simulink model "Modelo_MV_CIGRE_IPSD"  (R2019b)
settings: Solver=FixedStepAuto  StartTime=0.0  StopTime=0.3  FixedStep=Ts  RelTol=1e-3
PreLoadFcn:
  | r_1=0.501
  | l_1=0.716/(60*2*pi)
  | c_1=10e-6/(60*2*pi)
  | r_0=0.817
  | l_0=1.598 /(60*2*pi)
  | c_0=10e-6/(60*2*pi)
  | Sb=50e6
  | Ts=1e-4
InitFcn:
  | r_1=0.501;
  | l_1=0.716/(60*2*pi);
  | c_1=10e-6/(60*2*pi);
  | r_0=0.817;
  | l_0=1.598 /(60*2*pi);
  | c_0=10e-6/(60*2*pi);
  | Sb=50e6;
  | Ts=1e-4;
StartFcn:
  | r_1=0.501
  | l_1=0.716/(60*2*pi)
  | c_1=10e-6/(60*2*pi)
  | r_0=0.817
  | l_0=1.598 /(60*2*pi)
  | c_0=10e-6/(60*2*pi)
  | Sb=50e6
  | Ts=1e-5
undefined symbols (not defined in the file): D1, Delta
libraries: powerlib_meascontrol x112, powerlib x55, simulink x6
(part 2 of 3)

== system Modelo_MV_CIGRE_IPSD/DER1 ==
  Control IBRs : Subsystem
  Controlled Voltage Source : powerlib/Electrical Sources/Controlled Voltage Source  Initialize=on  Source_Type=AC  Amplitude=400*sqrt(2/3)  Phase=0  Frequency=60  Measurements=None
      settings: SourceProductName=Simscape Electrical
  Controlled Voltage Source2 : powerlib/Electrical Sources/Controlled Voltage Source  Initialize=on  Source_Type=AC  Amplitude=400*sqrt(2/3)  Phase=120  Frequency=60  Measurements=None
      settings: SourceProductName=Simscape Electrical
  Controlled Voltage Source3 : powerlib/Electrical Sources/Controlled Voltage Source  Initialize=on  Source_Type=AC  Amplitude=400*sqrt(2/3)  Phase=-120  Frequency=60  Measurements=None
      settings: SourceProductName=Simscape Electrical
  Ground : powerlib/Elements/Ground  LConnTagsString=a
      settings: SourceProductName=Simscape Electrical
  "Power (3ph, Instantaneous)" : powerlib_meascontrol/Measurements/Power (3ph, Instantaneous)
      settings: SourceProductName=Simscape Electrical
  Scope : Scope
  Scope1 : Scope  NumInputPorts=2
  Scope4 : Scope  NumInputPorts=3
  Scope5 : Scope
  Scope6 : Scope
  Three-Phase Series RLC Branch1 : powerlib/Elements/Three-Phase Series RLC Branch  LConnTagsString=A|B|C  RConnTagsString=A|B|C  BranchType=RL  Resistance=0.57  Inductance=1.5e-3  Capacitance=1e-6  Measurements=None
      settings: SourceProductName=Simscape Electrical
  Three-Phase Series RLC Branch2 : powerlib/Elements/Three-Phase Series RLC Branch  LConnTagsString=A|B|C  RConnTagsString=A|B|C  BranchType=C  Resistance=0.01  Inductance=1e-3  Capacitance=3e-6  Measurements=None
      settings: SourceProductName=Simscape Electrical
  Three-Phase V-I Measurement : powerlib/Measurements/Three-Phase V-I Measurement  VoltageMeasurement=phase-to-ground  SetLabelV=on  LabelV=Vabc_DER2  Vpu=on  VpuLL=off  CurrentMeasurement=yes  SetLabelI=on  LabelI=Iabc_DER2  Ipu=on  Pbase=100e3  Vbase=400  OutputType=Complex  PhasorSimulation=off  PSBequivalent=0
      settings: SourceProductName=Simscape Electrical
  Three-Phase Transformer Inductance Matrix Type (Two Windings) : powerlib/Elements/Three-Phase Transformer Inductance Matrix Type (Two Windings)  CoreType=Three single-phase cores  Winding1Connection=Yg  Winding2Connection=Delta (D1)  AutoTransformer=off  Measurements=None  NominalPower=[150e3, 60]  VLLnom=[20e3, 400]  WindingResistances=[0.01, 0.01]  NoLoadIexcPos=2  NoLoadPlossPos=1000  ShortCircuitReactancePos=0.06  ShortCircuitReactancePosAuto=0.06  NoLoadIexcZero=100  NoLoadPlossZero=1500  ShortCircuitReactanceZero=0.03  ShortCircuitReactanceZeroAuto=0.03
      settings: SourceProductName=Simscape Electrical  SourceProductBaseCode=PS
  A : PMIOPort  Side=Left
  B : PMIOPort  Port=2  Side=Left
  C : PMIOPort  Port=3  Side=Left
  wires:
  Control IBRs/2(Vb) -> Scope4/2, Controlled Voltage Source2/1
  [Vabc_DER2] -> "Power (3ph, Instantaneous)"/1, Scope/1, Scope1/2, Control IBRs/1(Vmeas)
  Control IBRs/3(Vc) -> Scope4/3, Controlled Voltage Source3/1
  "Power (3ph, Instantaneous)"/1 -> Scope5/1
  Control IBRs/1(Va) -> Scope4/1, Controlled Voltage Source/1
  "Power (3ph, Instantaneous)"/2 -> Scope6/1
  [Iabc_DER2] -> Scope1/1, "Power (3ph, Instantaneous)"/2, Control IBRs/2(Imeas)
  connections:
  Ground/LConn1 -- Three-Phase Series RLC Branch2/RConn1 -- Three-Phase Series RLC Branch2/RConn3 -- Controlled Voltage Source/LConn1 -- Controlled Voltage Source2/LConn1 -- Controlled Voltage Source3/LConn1 -- Three-Phase Series RLC Branch2/RConn2
  C/RConn1 -- Three-Phase Transformer Inductance Matrix Type (Two Windings)/LConn3
  Three-Phase Series RLC Branch1/RConn1 -- Controlled Voltage Source/RConn1
  Three-Phase Transformer Inductance Matrix Type (Two Windings)/RConn3 -- Three-Phase V-I Measurement/RConn3
  Three-Phase Transformer Inductance Matrix Type (Two Windings)/LConn2 -- B/RConn1
  Three-Phase Series RLC Branch1/LConn3 -- Three-Phase V-I Measurement/LConn3 -- Three-Phase Series RLC Branch2/LConn3
  Three-Phase Series RLC Branch1/RConn2 -- Controlled Voltage Source2/RConn1
  Three-Phase Series RLC Branch1/LConn1 -- Three-Phase V-I Measurement/LConn1 -- Three-Phase Series RLC Branch2/LConn1
  Three-Phase V-I Measurement/RConn1 -- Three-Phase Transformer Inductance Matrix Type (Two Windings)/RConn1
  Three-Phase V-I Measurement/RConn2 -- Three-Phase Transformer Inductance Matrix Type (Two Windings)/RConn2
  Three-Phase Series RLC Branch1/RConn3 -- Controlled Voltage Source3/RConn1
  Three-Phase Series RLC Branch1/LConn2 -- Three-Phase Series RLC Branch2/LConn2 -- Three-Phase V-I Measurement/LConn2
  A/RConn1 -- Three-Phase Transformer Inductance Matrix Type (Two Windings)/LConn1

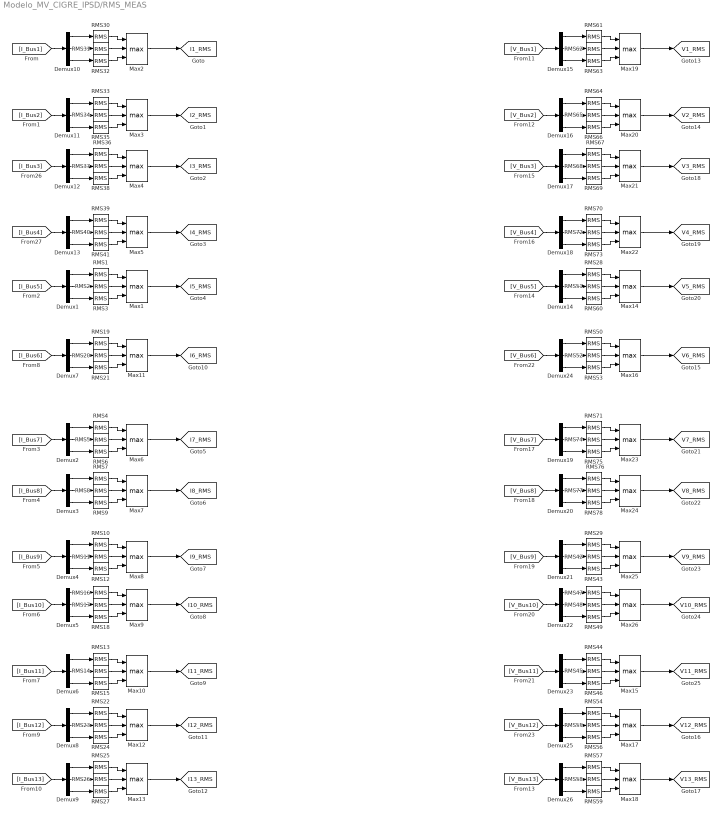
== system Modelo_MV_CIGRE_IPSD/RMS_MEAS ==
  Demux{1..26} (26 alike) : Demux  Outputs=3
  Max{1..26} (26 alike) : MinMax  Function=max  Inputs=3
  RMS{1..78} (78 alike) : powerlib_meascontrol/Measurements/RMS  TrueRMS=on  Freq=60  RMSInit=120  Ts=0
      settings: SourceProductName=Simscape Electrical
  tag scope: I10_RMS=global, I11_RMS=global, I12_RMS=global, I13_RMS=global, I1_RMS=global, I2_RMS=global, I3_RMS=global, I4_RMS=global, I5_RMS=global, I6_RMS=global, I7_RMS=global, I8_RMS=global, I9_RMS=global, V10_RMS=global, V11_RMS=global, V12_RMS=global, V13_RMS=global, V1_RMS=global, V2_RMS=global, V3_RMS=global, V4_RMS=global, V5_RMS=global, V6_RMS=global, V7_RMS=global, V8_RMS=global, V9_RMS=global
  wires:
  Demux10/3 -> RMS32/1
  RMS32/1 -> Max2/3
  RMS34/1 -> Max3/2
  RMS41/1 -> Max5/3
  RMS31/1 -> Max2/2
  Demux11/3 -> RMS35/1
  Demux10/1 -> RMS30/1
  [I_Bus1] -> Demux10/1
  Demux13/2 -> RMS40/1
  Demux12/2 -> RMS37/1
  Demux10/2 -> RMS31/1
  RMS35/1 -> Max3/3
  Demux11/2 -> RMS34/1
  RMS30/1 -> Max2/1
  [I_Bus2] -> Demux11/1
  Demux13/1 -> RMS39/1
  [I_Bus4] -> Demux13/1
  Demux11/1 -> RMS33/1
  RMS33/1 -> Max3/1
  RMS40/1 -> Max5/2
  Demux12/1 -> RMS36/1
  RMS36/1 -> Max4/1
  RMS37/1 -> Max4/2
  RMS39/1 -> Max5/1
  Demux13/3 -> RMS41/1
  RMS38/1 -> Max4/3
  [I_Bus3] -> Demux12/1
  Demux12/3 -> RMS38/1
  Demux3/3 -> RMS9/1
  [I_Bus8] -> Demux3/1
  RMS9/1 -> Max7/3
  Demux4/3 -> RMS12/1
  RMS10/1 -> Max8/1
  RMS8/1 -> Max7/2
  RMS7/1 -> Max7/1
  Demux3/1 -> RMS7/1
  RMS11/1 -> Max8/2
  RMS4/1 -> Max6/1
  Demux2/1 -> RMS4/1
  [I_Bus9] -> Demux4/1
  Demux4/1 -> RMS10/1
  [I_Bus7] -> Demux2/1
  RMS1/1 -> Max1/1
  Demux2/2 -> RMS5/1
  RMS6/1 -> Max6/3
  Demux1/2 -> RMS2/1
  Demux3/2 -> RMS8/1
  Demux4/2 -> RMS11/1
  [I_Bus5] -> Demux1/1
  Demux1/1 -> RMS1/1
  Demux2/3 -> RMS6/1
  RMS2/1 -> Max1/2
  RMS12/1 -> Max8/3
  RMS5/1 -> Max6/2
  RMS3/1 -> Max1/3
  Demux1/3 -> RMS3/1
  RMS15/1 -> Max10/3
  Demux6/2 -> RMS14/1
  Demux5/2 -> RMS17/1
  Demux6/1 -> RMS13/1
  [I_Bus11] -> Demux6/1
  RMS14/1 -> Max10/2
  Demux5/1 -> RMS16/1
  RMS16/1 -> Max9/1
  RMS17/1 -> Max9/2
  RMS13/1 -> Max10/1
  Demux6/3 -> RMS15/1
  RMS18/1 -> Max9/3
  [I_Bus10] -> Demux5/1
  Demux5/3 -> RMS18/1
  Max2/1 -> [I1_RMS]
  Max3/1 -> [I2_RMS]
  Max4/1 -> [I3_RMS]
  Max5/1 -> [I4_RMS]
  Max1/1 -> [I5_RMS]
  Max6/1 -> [I7_RMS]
  Max7/1 -> [I8_RMS]
  Max8/1 -> [I9_RMS]
  Max9/1 -> [I10_RMS]
  Max10/1 -> [I11_RMS]
  Max11/1 -> [I6_RMS]
  Demux7/3 -> RMS21/1
  RMS21/1 -> Max11/3
  RMS20/1 -> Max11/2
  Demux7/1 -> RMS19/1
  [I_Bus6] -> Demux7/1
  Demux7/2 -> RMS20/1
  RMS19/1 -> Max11/1
  Max12/1 -> [I12_RMS]
  Demux8/3 -> RMS24/1
  RMS22/1 -> Max12/1
  RMS23/1 -> Max12/2
  [I_Bus12] -> Demux8/1
  Demux8/1 -> RMS22/1
  Demux8/2 -> RMS23/1
  RMS24/1 -> Max12/3
  RMS27/1 -> Max13/3
  Demux9/2 -> RMS26/1
  Demux9/1 -> RMS25/1
  [I_Bus13] -> Demux9/1
  RMS26/1 -> Max13/2
  RMS25/1 -> Max13/1
  Demux9/3 -> RMS27/1
  Max13/1 -> [I13_RMS]
  Max18/1 -> [V13_RMS]
  Demux26/3 -> RMS59/1
  RMS57/1 -> Max18/1
  RMS58/1 -> Max18/2
  [V_Bus13] -> Demux26/1
  Demux26/1 -> RMS57/1
  Demux26/2 -> RMS58/1
  RMS59/1 -> Max18/3
  RMS56/1 -> Max17/3
  Demux25/2 -> RMS55/1
  Demux25/1 -> RMS54/1
  [V_Bus12] -> Demux25/1
  RMS55/1 -> Max17/2
  RMS54/1 -> Max17/1
  Demux25/3 -> RMS56/1
  Max17/1 -> [V12_RMS]
  RMS50/1 -> Max16/1
  Demux24/2 -> RMS52/1
  [V_Bus6] -> Demux24/1
  Demux24/1 -> RMS50/1
  RMS52/1 -> Max16/2
  RMS53/1 -> Max16/3
  Demux24/3 -> RMS53/1
  Max16/1 -> [V6_RMS]
  Max15/1 -> [V11_RMS]
  Max26/1 -> [V10_RMS]
  Max25/1 -> [V9_RMS]
  Max24/1 -> [V8_RMS]
  Max23/1 -> [V7_RMS]
  Max14/1 -> [V5_RMS]
  Max22/1 -> [V4_RMS]
  Max21/1 -> [V3_RMS]
  Max20/1 -> [V2_RMS]
  Max19/1 -> [V1_RMS]
  Demux22/3 -> RMS49/1
  [V_Bus10] -> Demux22/1
  RMS49/1 -> Max26/3
  Demux23/3 -> RMS46/1
  RMS44/1 -> Max15/1
  RMS48/1 -> Max26/2
  RMS47/1 -> Max26/1
  Demux22/1 -> RMS47/1
  RMS45/1 -> Max15/2
  [V_Bus11] -> Demux23/1
  Demux23/1 -> RMS44/1
  Demux22/2 -> RMS48/1
  Demux23/2 -> RMS45/1
  RMS46/1 -> Max15/3
  Demux14/3 -> RMS60/1
  RMS60/1 -> Max14/3
  RMS74/1 -> Max23/2
  RMS43/1 -> Max25/3
  RMS51/1 -> Max14/2
  Demux19/3 -> RMS75/1
  Demux14/1 -> RMS28/1
  [V_Bus5] -> Demux14/1
  Demux21/2 -> RMS42/1
  Demux20/2 -> RMS77/1
  Demux14/2 -> RMS51/1
  RMS75/1 -> Max23/3
  Demux19/2 -> RMS74/1
  RMS28/1 -> Max14/1
  [V_Bus7] -> Demux19/1
  Demux21/1 -> RMS29/1
  [V_Bus9] -> Demux21/1
  Demux19/1 -> RMS71/1
  RMS71/1 -> Max23/1
  RMS42/1 -> Max25/2
  Demux20/1 -> RMS76/1
  RMS76/1 -> Max24/1
  RMS77/1 -> Max24/2
  RMS29/1 -> Max25/1
  Demux21/3 -> RMS43/1
  RMS78/1 -> Max24/3
  [V_Bus8] -> Demux20/1
  Demux20/3 -> RMS78/1
  Demux17/3 -> RMS69/1
  [V_Bus3] -> Demux17/1
  RMS69/1 -> Max21/3
  Demux18/3 -> RMS73/1
  RMS70/1 -> Max22/1
  RMS68/1 -> Max21/2
  RMS67/1 -> Max21/1
  Demux17/1 -> RMS67/1
  RMS72/1 -> Max22/2
  RMS64/1 -> Max20/1
  Demux16/1 -> RMS64/1
  [V_Bus4] -> Demux18/1
  Demux18/1 -> RMS70/1
  [V_Bus2] -> Demux16/1
  RMS61/1 -> Max19/1
  Demux16/2 -> RMS65/1
  RMS66/1 -> Max20/3
  Demux15/2 -> RMS62/1
  Demux17/2 -> RMS68/1
  Demux18/2 -> RMS72/1
  [V_Bus1] -> Demux15/1
  Demux15/1 -> RMS61/1
  Demux16/3 -> RMS66/1
  RMS62/1 -> Max19/2
  RMS73/1 -> Max22/3
  RMS65/1 -> Max20/2
  RMS63/1 -> Max19/3
  Demux15/3 -> RMS63/1

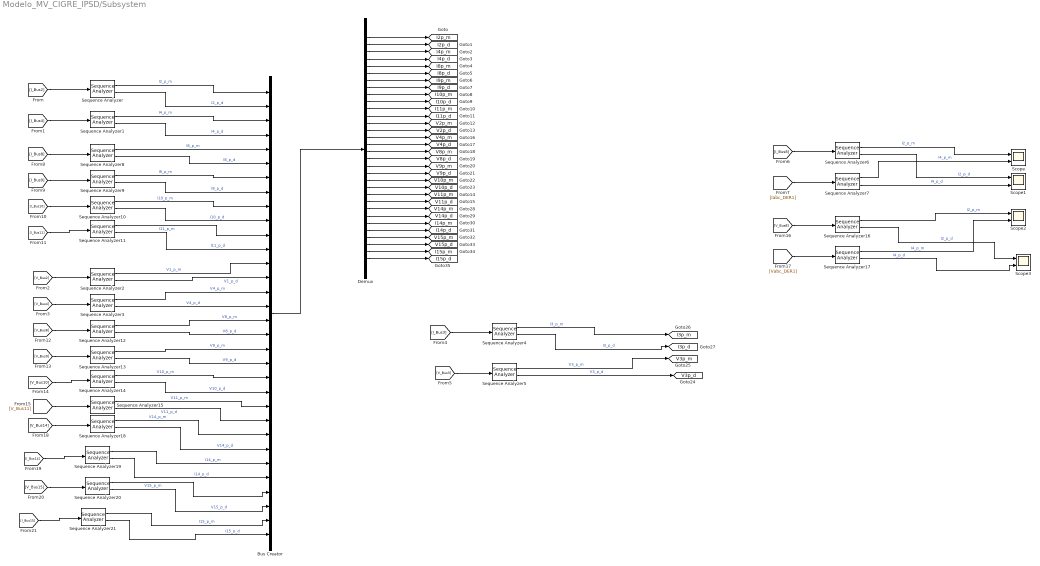
== system Modelo_MV_CIGRE_IPSD/Subsystem ==
  Bus Creator : BusCreator  Inputs=32
  Demux : Demux  Outputs=32
  Scope{,1..3} (4 alike) : Scope  NumInputPorts=2
  Sequence Analyzer{,1..5,8..15,18..21} (18 alike) : powerlib_meascontrol/Measurements/Sequence Analyzer  Freq=60  n=1  seq=Positive  InInit=[ 1 0]  Ts=Ts
      settings: SourceProductName=Simscape Electrical  SourceProductBaseCode=PS
  Sequence Analyzer{6..7,16..17} (4 alike) : powerlib_meascontrol/Measurements/Sequence Analyzer  Freq=60  n=1  seq=Positive Negative Zero  InInit=[ 1 0]  Ts=Ts
      settings: SourceProductName=Simscape Electrical  SourceProductBaseCode=PS
  tag scope: I10p_d=global, I10p_m=global, I11p_d=global, I11p_m=global, I14p_d=global, I14p_m=global, I15p_d=global, I15p_m=global, I2p_d=global, I2p_m=global, I3p_d=global, I3p_m=global, I4p_d=global, I4p_m=global, I8p_d=global, I8p_m=global, I9p_d=global, I9p_m=global, V10p_d=global, V10p_m=global, V11p_d=global, V11p_m=global, V14p_d=global, V14p_m=global, V15p_d=global, V15p_m=global, V2p_d=global, V2p_m=global, V3p_d=global, V3p_m=global, V4p_d=global, V4p_m=global, V8p_d=global, V8p_m=global, V9p_d=global, V9p_m=global
  wires:
  [I_Bus2] -> Sequence Analyzer/1
  [I_Bus4] -> Sequence Analyzer1/1
  [V_Bus4] -> Sequence Analyzer3/1
  [V_Bus2] -> Sequence Analyzer2/1
  Sequence Analyzer/1 -> Bus Creator/1  "I2_p_m"
  Sequence Analyzer/2 -> Bus Creator/2  "I2_p_d"
  Sequence Analyzer1/1 -> Bus Creator/3  "I4_p_m"
  Sequence Analyzer1/2 -> Bus Creator/4  "I4_p_d"
  Sequence Analyzer2/1 -> Bus Creator/13  "V1_p_m"
  Sequence Analyzer2/2 -> Bus Creator/14  "V1_p_d"
  Sequence Analyzer3/1 -> Bus Creator/15  "V4_p_m"
  Sequence Analyzer3/2 -> Bus Creator/16  "V4_p_d"
  Bus Creator/1 -> Demux/1
  Sequence Analyzer8/2 -> Bus Creator/6  "I8_p_d"
  Sequence Analyzer8/1 -> Bus Creator/5  "I8_p_m"
  [I_Bus8] -> Sequence Analyzer8/1
  [I_Bus9] -> Sequence Analyzer9/1
  Sequence Analyzer9/1 -> Bus Creator/7  "I9_p_m"
  Sequence Analyzer9/2 -> Bus Creator/8  "I9_p_d"
  Sequence Analyzer10/2 -> Bus Creator/10  "I10_p_d"
  Sequence Analyzer10/1 -> Bus Creator/9  "I10_p_m"
  [I_Bus10] -> Sequence Analyzer10/1
  [I_Bus11] -> Sequence Analyzer11/1
  Sequence Analyzer11/1 -> Bus Creator/11  "I11_p_m"
  Sequence Analyzer11/2 -> Bus Creator/12  "I11_p_d"
  Sequence Analyzer13/2 -> Bus Creator/20  "V9_p_d"
  Sequence Analyzer13/1 -> Bus Creator/19  "V9_p_m"
  Sequence Analyzer12/2 -> Bus Creator/18  "V8_p_d"
  Sequence Analyzer12/1 -> Bus Creator/17  "V8_p_m"
  [V_Bus8] -> Sequence Analyzer12/1
  [V_Bus9] -> Sequence Analyzer13/1
  [V_Bus11] -> Sequence Analyzer15/1
  [V_Bus10] -> Sequence Analyzer14/1
  Sequence Analyzer14/1 -> Bus Creator/21  "V10_p_m"
  Sequence Analyzer14/2 -> Bus Creator/22  "V10_p_d"
  Sequence Analyzer15/1 -> Bus Creator/23  "V11_p_m"
  Sequence Analyzer15/2 -> Bus Creator/24  "V11_p_d"
  Demux/1 -> [I2p_m]
  Demux/2 -> [I2p_d]
  Demux/3 -> [I4p_m]
  Demux/4 -> [I4p_d]
  Demux/5 -> [I8p_m]
  Demux/6 -> [I8p_d]
  Demux/7 -> [I9p_m]
  Demux/8 -> [I9p_d]
  Demux/9 -> [I10p_m]
  Demux/10 -> [I10p_d]
  Demux/11 -> [I11p_m]
  Demux/12 -> [I11p_d]
  Demux/13 -> [V2p_m]
  Demux/14 -> [V2p_d]
  Demux/15 -> [V4p_m]
  Demux/16 -> [V4p_d]
  Demux/17 -> [V8p_m]
  Demux/18 -> [V8p_d]
  Demux/19 -> [V9p_m]
  Demux/20 -> [V9p_d]
  Demux/21 -> [V10p_m]
  Demux/22 -> [V10p_d]
  Demux/23 -> [V11p_m]
  Demux/24 -> [V11p_d]
  Sequence Analyzer4/1 -> [I3p_m]  "I3_p_m"
  Sequence Analyzer4/2 -> [I3p_d]  "I3_p_d"
  [I_Bus3] -> Sequence Analyzer4/1
  Sequence Analyzer5/2 -> [V3p_d]  "V3_p_d"
  Sequence Analyzer5/1 -> [V3p_m]  "V3_p_m"
  [V_Bus3] -> Sequence Analyzer5/1
  Sequence Analyzer6/1 -> Scope/1  "I2_p_m"
  [Iabc_DER1] -> Sequence Analyzer7/1
  Sequence Analyzer7/1 -> Scope/2  "I4_p_m"
  Sequence Analyzer6/2 -> Scope1/1  "I2_p_d"
  [I_Bus8] -> Sequence Analyzer6/1
  Sequence Analyzer7/2 -> Scope1/2  "I4_p_d"
  Sequence Analyzer17/2 -> Scope3/2  "I4_p_d"
  [V_Bus8] -> Sequence Analyzer16/1
  Sequence Analyzer16/2 -> Scope3/1  "I2_p_d"
  Sequence Analyzer17/1 -> Scope2/2  "I4_p_m"
  [Vabc_DER1] -> Sequence Analyzer17/1
  Sequence Analyzer16/1 -> Scope2/1  "I2_p_m"
  Sequence Analyzer18/2 -> Bus Creator/26  "V14_p_d"
  Sequence Analyzer18/1 -> Bus Creator/25  "V14_p_m"
  [V_Bus14] -> Sequence Analyzer18/1
  Demux/25 -> [V14p_m]
  Demux/26 -> [V14p_d]
  Sequence Analyzer19/2 -> Bus Creator/28  "I14_p_d"
  Sequence Analyzer19/1 -> Bus Creator/27  "I14_p_m"
  [I_Bus14] -> Sequence Analyzer19/1
  Demux/27 -> [I14p_m]
  Demux/28 -> [I14p_d]
  [I_Bus15] -> Sequence Analyzer21/1
  Sequence Analyzer21/1 -> Bus Creator/31  "I15_p_m"
  Sequence Analyzer21/2 -> Bus Creator/32  "I15_p_d"
  [V_Bus15] -> Sequence Analyzer20/1
  Sequence Analyzer20/1 -> Bus Creator/29  "V15_p_m"
  Sequence Analyzer20/2 -> Bus Creator/30  "V15_p_d"
  Demux/29 -> [V15p_m]
  Demux/30 -> [V15p_d]
  Demux/31 -> [I15p_m]
  Demux/32 -> [I15p_d]

== system Modelo_MV_CIGRE_IPSD/Subsystem1 ==
  Bus Creator : BusCreator  Inputs=9
  Demux : Demux  Outputs=5
  Demux1 : Demux
  Scope : Scope
  To File : ToFile  Filename=Disparos.mat  MatrixName=FaultF7_ISL  SaveFormat=Timeseries
  wires:
  Bus Creator/1 -> Scope/1, To File/1
  [Disparos_1] -> Demux/1
  Demux/1 -> Bus Creator/1  "t8"
  Demux/2 -> Bus Creator/2  "t10"
  Demux/3 -> Bus Creator/3  "t9"
  Demux/4 -> Bus Creator/4  "t11"
  [Disparos2] -> Demux1/1
  Demux/5 -> Bus Creator/5  "t14"
  Demux1/1 -> Bus Creator/6  "t2"
  Demux1/2 -> Bus Creator/7  "t3"
  Demux1/3 -> Bus Creator/8  "t4"
  Demux1/4 -> Bus Creator/9  "t15"

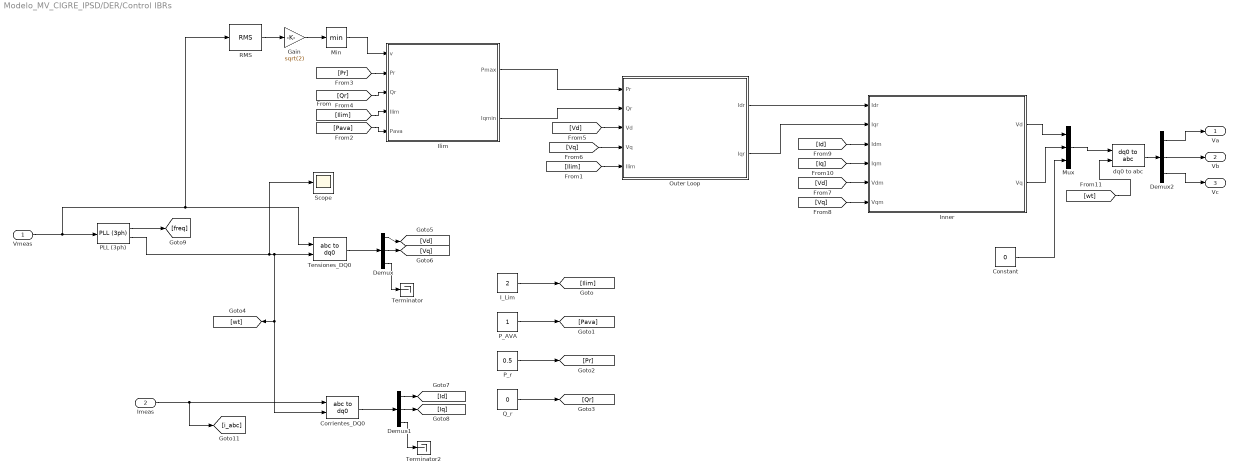
== system Modelo_MV_CIGRE_IPSD/DER/Control IBRs ==
  Vmeas : Inport
  Imeas : Inport  Port=2
  Constant : Constant  Value=0
  Corrientes_DQ0 : powerlib_meascontrol/Transformations/abc to dq0  Alignment=90 degrees behind phase A axis
      settings: SourceProductName=Simscape Electrical
  Demux : Demux  Outputs=3
  Demux1 : Demux  Outputs=3
  Demux2 : Demux  Outputs=3
  Gain : Gain  Gain=sqrt(2)
  I_Lim : Constant  Value=2
  Ilim : MATLAB Function  TreatAsAtomicUnit=on
  Inner : Subsystem
  Min : MinMax
  Mux : Mux  Inputs=3
  Outer Loop : MATLAB Function  TreatAsAtomicUnit=on
  PLL (3ph) : powerlib_meascontrol/PLL/PLL (3ph)  Fmin=55  Par_Init=[0, 60]  ParK=[50,25, 0]  TcD=1e-4  MaxRateChangeFreq=12  FilterCutOffFreq=25  Ts=0  AGC=on
      settings: SourceProductName=Simscape Electrical
  P_AVA : Constant
  P_r : Constant  Value=0.5
  Q_r : Constant  Value=0
  RMS : powerlib_meascontrol/Measurements/RMS  TrueRMS=on  Freq=60  RMSInit=1  Ts=0
      settings: SourceProductName=Simscape Electrical
  Scope : Scope
  Tensiones_DQ0 : powerlib_meascontrol/Transformations/abc to dq0  Alignment=90 degrees behind phase A axis
      settings: SourceProductName=Simscape Electrical
  Terminator : Terminator
  Terminator2 : Terminator
  dq0 to abc : powerlib_meascontrol/Transformations/dq0 to abc  Alignment=90 degrees behind phase A axis
      settings: SourceProductName=Simscape Electrical
  Va : Outport
  Vb : Outport  Port=2
  Vc : Outport  Port=3
  wires:
  Tensiones_DQ0/1 -> Demux/1
  Outer Loop/2(Iqr) -> Inner/2(Iqr)
  dq0 to abc/1 -> Demux2/1
  [Qr] -> Ilim/3(Qr)
  [Ilim] -> Ilim/4(Ilim)
  Demux1/1 -> [Id]
  Ilim/1(Pmax) -> Outer Loop/1(Pr)
  [Vq] -> Inner/6(Vqm)
  [Vd] -> Inner/5(Vdm)
  [Iq] -> Inner/4(Iqm)
  Demux1/3 -> Terminator2/1
  Demux/1 -> [Vd]
  [Id] -> Inner/3(Idm)
  [Vd] -> Outer Loop/3(Vd)
  [Pr] -> Ilim/2(Pr)
  P_AVA/1 -> [Pava]
  I_Lim/1 -> [Ilim]
  P_r/1 -> [Pr]
  Q_r/1 -> [Qr]
  Outer Loop/1(Idr) -> Inner/1(Idr)
  [Vq] -> Outer Loop/4(Vq)
  [Pava] -> Ilim/5(Pava)
  Inner/1(Vd) -> Mux/1
  [wt] -> dq0 to abc/2
  Constant/1 -> Mux/3
  Ilim/2(Iqmin) -> Outer Loop/2(Qr)
  Demux/2 -> [Vq]
  Mux/1 -> dq0 to abc/1
  Demux/3 -> Terminator/1
  [Ilim] -> Outer Loop/5(Ilim)
  Inner/2(Vq) -> Mux/2
  Corrientes_DQ0/1 -> Demux1/1
  Demux1/2 -> [Iq]
  Vmeas/1 -> RMS/1, Tensiones_DQ0/1, PLL (3ph)/1
  Imeas/1 -> [i_abc], Corrientes_DQ0/1
  Demux2/1 -> Va/1
  Demux2/2 -> Vb/1
  Demux2/3 -> Vc/1
  Min/1 -> Ilim/1(v)
  RMS/1 -> Gain/1
  Gain/1 -> Min/1
  PLL (3ph)/1 -> [freq]
  PLL (3ph)/2 -> Scope/1, Corrientes_DQ0/2, [wt], Tensiones_DQ0/2

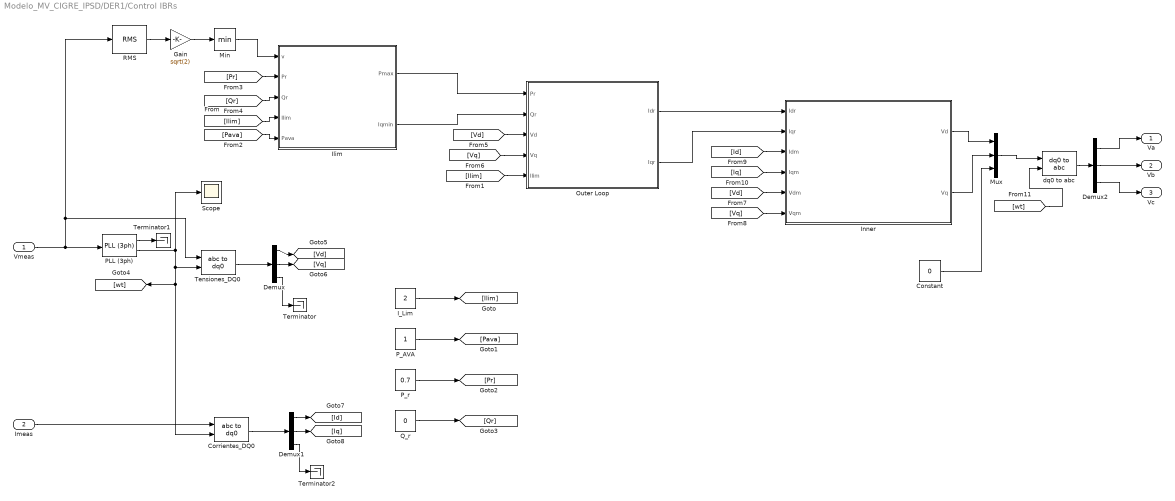
== system Modelo_MV_CIGRE_IPSD/DER1/Control IBRs ==
  Vmeas : Inport
  Imeas : Inport  Port=2
  Constant : Constant  Value=0
  Corrientes_DQ0 : powerlib_meascontrol/Transformations/abc to dq0  Alignment=90 degrees behind phase A axis
      settings: SourceProductName=Simscape Electrical
  Demux : Demux  Outputs=3
  Demux1 : Demux  Outputs=3
  Demux2 : Demux  Outputs=3
  Gain : Gain  Gain=sqrt(2)
  I_Lim : Constant  Value=2
  Ilim : MATLAB Function  TreatAsAtomicUnit=on
  Inner : Subsystem
  Min : MinMax
  Mux : Mux  Inputs=3
  Outer Loop : MATLAB Function  TreatAsAtomicUnit=on
  PLL (3ph) : powerlib_meascontrol/PLL/PLL (3ph)  Fmin=55  Par_Init=[0, 60]  ParK=[50,25, 0]  TcD=1e-4  MaxRateChangeFreq=12  FilterCutOffFreq=25  Ts=0  AGC=on
      settings: SourceProductName=Simscape Electrical
  P_AVA : Constant
  P_r : Constant  Value=0.7
  Q_r : Constant  Value=0
  RMS : powerlib_meascontrol/Measurements/RMS  TrueRMS=on  Freq=60  RMSInit=1  Ts=0
      settings: SourceProductName=Simscape Electrical
  Scope : Scope
  Tensiones_DQ0 : powerlib_meascontrol/Transformations/abc to dq0  Alignment=90 degrees behind phase A axis
      settings: SourceProductName=Simscape Electrical
  Terminator : Terminator
  Terminator1 : Terminator
  Terminator2 : Terminator
  dq0 to abc : powerlib_meascontrol/Transformations/dq0 to abc  Alignment=90 degrees behind phase A axis
      settings: SourceProductName=Simscape Electrical
  Va : Outport
  Vb : Outport  Port=2
  Vc : Outport  Port=3
  wires:
  Tensiones_DQ0/1 -> Demux/1
  Outer Loop/2(Iqr) -> Inner/2(Iqr)
  dq0 to abc/1 -> Demux2/1
  [Qr] -> Ilim/3(Qr)
  [Ilim] -> Ilim/4(Ilim)
  Demux1/1 -> [Id]
  Ilim/1(Pmax) -> Outer Loop/1(Pr)
  [Vq] -> Inner/6(Vqm)
  [Vd] -> Inner/5(Vdm)
  [Iq] -> Inner/4(Iqm)
  Demux1/3 -> Terminator2/1
  Demux/1 -> [Vd]
  [Id] -> Inner/3(Idm)
  [Vd] -> Outer Loop/3(Vd)
  [Pr] -> Ilim/2(Pr)
  P_AVA/1 -> [Pava]
  PLL (3ph)/2 -> Scope/1, Corrientes_DQ0/2, [wt], Tensiones_DQ0/2
  I_Lim/1 -> [Ilim]
  P_r/1 -> [Pr]
  Q_r/1 -> [Qr]
  Outer Loop/1(Idr) -> Inner/1(Idr)
  [Vq] -> Outer Loop/4(Vq)
  [Pava] -> Ilim/5(Pava)
  Inner/1(Vd) -> Mux/1
  [wt] -> dq0 to abc/2
  Constant/1 -> Mux/3
  Ilim/2(Iqmin) -> Outer Loop/2(Qr)
  Demux/2 -> [Vq]
  Mux/1 -> dq0 to abc/1
  Demux/3 -> Terminator/1
  [Ilim] -> Outer Loop/5(Ilim)
  Inner/2(Vq) -> Mux/2
  Corrientes_DQ0/1 -> Demux1/1
  Demux1/2 -> [Iq]
  Vmeas/1 -> RMS/1, Tensiones_DQ0/1, PLL (3ph)/1
  Imeas/1 -> Corrientes_DQ0/1
  PLL (3ph)/1 -> Terminator1/1
  Demux2/1 -> Va/1
  Demux2/2 -> Vb/1
  Demux2/3 -> Vc/1
  Min/1 -> Ilim/1(v)
  RMS/1 -> Gain/1
  Gain/1 -> Min/1

== system Modelo_MV_CIGRE_IPSD/DER/Control IBRs/Inner ==
  Idr : Inport
  Iqr : Inport  Port=2
  Idm : Inport  Port=3
  Iqm : Inport  Port=4
  Vdm : Inport  Port=5
  Vqm : Inport  Port=6
  Add : Sum  Inputs=+++-
  Add1 : Sum  Inputs=++++
  Delay : Delay  DelayLength=1  InitialCondition=0
  Delay1 : Delay  DelayLength=1  InitialCondition=0
  Gain : Gain  Gain=1/1.6
  Gain1 : Gain  Gain=1/1.6
  Gain2 : Gain  Gain=400*sqrt(2/3)
  Gain3 : Gain  Gain=400*sqrt(2/3)
  Lf : Constant  Value=1.5e-3*2*pi*60
  PID Controller : simulink/Continuous/PID Controller  Controller=PI  Form=Parallel  TimeDomain=Discrete-time  SampleTime=-1  IntegratorMethod=Forward Euler  FilterMethod=Forward Euler  ControllerParametersSource=internal  P=0.70  I=50  D=0  UseFilter=on  N=100  TunerSelectOption=Transfer Function Based (PID Tuner App)  InitialConditionSource=internal  InitialConditionForIntegrator=0  InitialConditionForFilter=0  DifferentiatorICPrevScaledInput=0  ExternalReset=none  TrackingMode=off  Kt=1  LimitOutput=off  UpperSaturationLimit=inf  LowerSaturationLimit=-inf  LinearizeAsGain=on  AntiWindupMode=none  Kb=1  POutMin=[]  POutMax=[]  IOutMin=[]  IOutMax=[]  DOutMin=[]  DOutMax=[]  NOutMin=[]  NOutMax=[]  SumOutMin=[]  SumOutMax=[]  SaturationOutMin=[]  SaturationOutMax=[]  PParamMin=[]  PParamMax=[]  IParamMin=[]  IParamMax=[]  DParamMin=[]  DParamMax=[]  NParamMin=[]  NParamMax=[]  KbParamMin=[]  KbParamMax=[]  KtParamMin=[]  KtParamMax=[]  KbOutMin=[]  KbOutMax=[]  KtOutMin=[]  KtOutMax=[]  IntegratorOutMin=[]  IntegratorOutMax=[]  FilterOutMin=[]  FilterOutMax=[]  SumI1OutMin=[]  SumI1OutMax=[]  SumI2OutMin=[]  SumI2OutMax=[]  SumI3OutMin=[]  SumI3OutMax=[]  SumI4OutMin=[]  SumI4OutMax=[]  SumDOutMin=[]  SumDOutMax=[]  DifferentiatorOutMin=[]  DifferentiatorOutMax=[]  FilterDiffOutCoefMin=[]  FilterDiffOutCoefMax=[]  ReciprocalOutMin=[]  ReciprocalOutMax=[]  SumDenOutMin=[]  SumDenOutMax=[]  SumNumOutMin=[]  SumNumOutMax=[]  DivideOutMin=[]  DivideOutMax=[]  IntegratorContinuousStateAttributes=''  IntegratorStateMustResolveToSignalObject=off  IntegratorRTWStateStorageClass=Auto  FilterContinuousStateAttributes=''  FilterStateMustResolveToSignalObject=off  FilterRTWStateStorageClass=Auto  ParallelPVariant=InternalParameters  IdealPVariant=Disabled  IVariant=InternalParameters  DVariant=Disabled  IntegratorVariant=Discrete  SatVariant=Disabled  AWVariant=Passthrough  PCopyVariant=Disabled  TRVariant=Disabled  FdbkBlocksVariant=Forward  IdealPFdbkVariant=Disabled  SatFdbkVariant=Disabled  DerivativeFilterVariant=Disabled  NVariant=Disabled  NCopyVariant=Disabled_SignalSpec  FilterICVariant=Disabled  IntegratorICVariant=InternalICs  ExternalResetVariant=Disabled  TRSumVariant=Passthrough  SumFdbkVariant=Disabled  SumVariant=Sum_PI
  PID Controller1 : simulink/Continuous/PID Controller  Controller=PI  Form=Parallel  TimeDomain=Discrete-time  SampleTime=-1  IntegratorMethod=Forward Euler  FilterMethod=Forward Euler  ControllerParametersSource=internal  P=0.7  I=50  D=0  UseFilter=on  N=100  TunerSelectOption=Transfer Function Based (PID Tuner App)  InitialConditionSource=internal  InitialConditionForIntegrator=0  InitialConditionForFilter=0  DifferentiatorICPrevScaledInput=0  ExternalReset=none  TrackingMode=off  Kt=1  LimitOutput=off  UpperSaturationLimit=inf  LowerSaturationLimit=-inf  LinearizeAsGain=on  AntiWindupMode=none  Kb=1  POutMin=[]  POutMax=[]  IOutMin=[]  IOutMax=[]  DOutMin=[]  DOutMax=[]  NOutMin=[]  NOutMax=[]  SumOutMin=[]  SumOutMax=[]  SaturationOutMin=[]  SaturationOutMax=[]  PParamMin=[]  PParamMax=[]  IParamMin=[]  IParamMax=[]  DParamMin=[]  DParamMax=[]  NParamMin=[]  NParamMax=[]  KbParamMin=[]  KbParamMax=[]  KtParamMin=[]  KtParamMax=[]  KbOutMin=[]  KbOutMax=[]  KtOutMin=[]  KtOutMax=[]  IntegratorOutMin=[]  IntegratorOutMax=[]  FilterOutMin=[]  FilterOutMax=[]  SumI1OutMin=[]  SumI1OutMax=[]  SumI2OutMin=[]  SumI2OutMax=[]  SumI3OutMin=[]  SumI3OutMax=[]  SumI4OutMin=[]  SumI4OutMax=[]  SumDOutMin=[]  SumDOutMax=[]  DifferentiatorOutMin=[]  DifferentiatorOutMax=[]  FilterDiffOutCoefMin=[]  FilterDiffOutCoefMax=[]  ReciprocalOutMin=[]  ReciprocalOutMax=[]  SumDenOutMin=[]  SumDenOutMax=[]  SumNumOutMin=[]  SumNumOutMax=[]  DivideOutMin=[]  DivideOutMax=[]  IntegratorContinuousStateAttributes=''  IntegratorStateMustResolveToSignalObject=off  IntegratorRTWStateStorageClass=Auto  FilterContinuousStateAttributes=''  FilterStateMustResolveToSignalObject=off  FilterRTWStateStorageClass=Auto  ParallelPVariant=InternalParameters  IdealPVariant=Disabled  IVariant=InternalParameters  DVariant=Disabled  IntegratorVariant=Discrete  SatVariant=Disabled  AWVariant=Passthrough  PCopyVariant=Disabled  TRVariant=Disabled  FdbkBlocksVariant=Forward  IdealPFdbkVariant=Disabled  SatFdbkVariant=Disabled  DerivativeFilterVariant=Disabled  NVariant=Disabled  NCopyVariant=Disabled_SignalSpec  FilterICVariant=Disabled  IntegratorICVariant=InternalICs  ExternalResetVariant=Disabled  TRSumVariant=Passthrough  SumFdbkVariant=Disabled  SumVariant=Sum_PI
  Product{,1..4} (5 alike) : Product
  Rf : Constant  Value=0.57
  Sum : Sum  Inputs=|+-
  Sum1 : Sum  Inputs=|+-
  Vd : Outport
  Vq : Outport  Port=2
  wires:
  Idr/1 -> Sum/1
  Idm/1 -> Product/1, Product4/1, Sum/2
  Iqr/1 -> Sum1/1
  Iqm/1 -> Product3/1, Sum1/2
  Sum/1 -> PID Controller/1
  Sum1/1 -> PID Controller1/1
  Gain3/1 -> Vq/1
  Add/1 -> Delay/1
  Vdm/1 -> Add/1
  Product/1 -> Add/3
  Rf/1 -> Gain/1
  Gain/1 -> Product1/2, Product/2
  Lf/1 -> Gain1/1
  PID Controller/1 -> Product1/1
  Product1/1 -> Add/2
  PID Controller1/1 -> Product2/1
  Gain1/1 -> Product4/2, Product3/2, Product2/2
  Gain2/1 -> Vd/1
  Add1/1 -> Delay1/1
  Vqm/1 -> Add1/2
  Product3/1 -> Add1/3, Add/4
  Product2/1 -> Add1/1
  Product4/1 -> Add1/4
  Delay/1 -> Gain2/1
  Delay1/1 -> Gain3/1

== system Modelo_MV_CIGRE_IPSD/DER1/Control IBRs/Inner ==
  Idr : Inport
  Iqr : Inport  Port=2
  Idm : Inport  Port=3
  Iqm : Inport  Port=4
  Vdm : Inport  Port=5
  Vqm : Inport  Port=6
  Add : Sum  Inputs=+++-
  Add1 : Sum  Inputs=++++
  Delay : Delay  DelayLength=1  InitialCondition=0
  Delay1 : Delay  DelayLength=1  InitialCondition=0
  Gain : Gain  Gain=1/1.6
  Gain1 : Gain  Gain=1/1.6
  Gain2 : Gain  Gain=400*sqrt(2/3)
  Gain3 : Gain  Gain=400*sqrt(2/3)
  Lf : Constant  Value=1.5e-3*2*pi*60
  PID Controller : simulink/Continuous/PID Controller  Controller=PI  Form=Parallel  TimeDomain=Discrete-time  SampleTime=-1  IntegratorMethod=Forward Euler  FilterMethod=Forward Euler  ControllerParametersSource=internal  P=0.70  I=50  D=0  UseFilter=on  N=100  TunerSelectOption=Transfer Function Based (PID Tuner App)  InitialConditionSource=internal  InitialConditionForIntegrator=0  InitialConditionForFilter=0  DifferentiatorICPrevScaledInput=0  ExternalReset=none  TrackingMode=off  Kt=1  LimitOutput=off  UpperSaturationLimit=inf  LowerSaturationLimit=-inf  LinearizeAsGain=on  AntiWindupMode=none  Kb=1  POutMin=[]  POutMax=[]  IOutMin=[]  IOutMax=[]  DOutMin=[]  DOutMax=[]  NOutMin=[]  NOutMax=[]  SumOutMin=[]  SumOutMax=[]  SaturationOutMin=[]  SaturationOutMax=[]  PParamMin=[]  PParamMax=[]  IParamMin=[]  IParamMax=[]  DParamMin=[]  DParamMax=[]  NParamMin=[]  NParamMax=[]  KbParamMin=[]  KbParamMax=[]  KtParamMin=[]  KtParamMax=[]  KbOutMin=[]  KbOutMax=[]  KtOutMin=[]  KtOutMax=[]  IntegratorOutMin=[]  IntegratorOutMax=[]  FilterOutMin=[]  FilterOutMax=[]  SumI1OutMin=[]  SumI1OutMax=[]  SumI2OutMin=[]  SumI2OutMax=[]  SumI3OutMin=[]  SumI3OutMax=[]  SumI4OutMin=[]  SumI4OutMax=[]  SumDOutMin=[]  SumDOutMax=[]  DifferentiatorOutMin=[]  DifferentiatorOutMax=[]  FilterDiffOutCoefMin=[]  FilterDiffOutCoefMax=[]  ReciprocalOutMin=[]  ReciprocalOutMax=[]  SumDenOutMin=[]  SumDenOutMax=[]  SumNumOutMin=[]  SumNumOutMax=[]  DivideOutMin=[]  DivideOutMax=[]  IntegratorContinuousStateAttributes=''  IntegratorStateMustResolveToSignalObject=off  IntegratorRTWStateStorageClass=Auto  FilterContinuousStateAttributes=''  FilterStateMustResolveToSignalObject=off  FilterRTWStateStorageClass=Auto  ParallelPVariant=InternalParameters  IdealPVariant=Disabled  IVariant=InternalParameters  DVariant=Disabled  IntegratorVariant=Discrete  SatVariant=Disabled  AWVariant=Passthrough  PCopyVariant=Disabled  TRVariant=Disabled  FdbkBlocksVariant=Forward  IdealPFdbkVariant=Disabled  SatFdbkVariant=Disabled  DerivativeFilterVariant=Disabled  NVariant=Disabled  NCopyVariant=Disabled_SignalSpec  FilterICVariant=Disabled  IntegratorICVariant=InternalICs  ExternalResetVariant=Disabled  TRSumVariant=Passthrough  SumFdbkVariant=Disabled  SumVariant=Sum_PI
  PID Controller1 : simulink/Continuous/PID Controller  Controller=PI  Form=Parallel  TimeDomain=Discrete-time  SampleTime=-1  IntegratorMethod=Forward Euler  FilterMethod=Forward Euler  ControllerParametersSource=internal  P=0.7  I=50  D=0  UseFilter=on  N=100  TunerSelectOption=Transfer Function Based (PID Tuner App)  InitialConditionSource=internal  InitialConditionForIntegrator=0  InitialConditionForFilter=0  DifferentiatorICPrevScaledInput=0  ExternalReset=none  TrackingMode=off  Kt=1  LimitOutput=off  UpperSaturationLimit=inf  LowerSaturationLimit=-inf  LinearizeAsGain=on  AntiWindupMode=none  Kb=1  POutMin=[]  POutMax=[]  IOutMin=[]  IOutMax=[]  DOutMin=[]  DOutMax=[]  NOutMin=[]  NOutMax=[]  SumOutMin=[]  SumOutMax=[]  SaturationOutMin=[]  SaturationOutMax=[]  PParamMin=[]  PParamMax=[]  IParamMin=[]  IParamMax=[]  DParamMin=[]  DParamMax=[]  NParamMin=[]  NParamMax=[]  KbParamMin=[]  KbParamMax=[]  KtParamMin=[]  KtParamMax=[]  KbOutMin=[]  KbOutMax=[]  KtOutMin=[]  KtOutMax=[]  IntegratorOutMin=[]  IntegratorOutMax=[]  FilterOutMin=[]  FilterOutMax=[]  SumI1OutMin=[]  SumI1OutMax=[]  SumI2OutMin=[]  SumI2OutMax=[]  SumI3OutMin=[]  SumI3OutMax=[]  SumI4OutMin=[]  SumI4OutMax=[]  SumDOutMin=[]  SumDOutMax=[]  DifferentiatorOutMin=[]  DifferentiatorOutMax=[]  FilterDiffOutCoefMin=[]  FilterDiffOutCoefMax=[]  ReciprocalOutMin=[]  ReciprocalOutMax=[]  SumDenOutMin=[]  SumDenOutMax=[]  SumNumOutMin=[]  SumNumOutMax=[]  DivideOutMin=[]  DivideOutMax=[]  IntegratorContinuousStateAttributes=''  IntegratorStateMustResolveToSignalObject=off  IntegratorRTWStateStorageClass=Auto  FilterContinuousStateAttributes=''  FilterStateMustResolveToSignalObject=off  FilterRTWStateStorageClass=Auto  ParallelPVariant=InternalParameters  IdealPVariant=Disabled  IVariant=InternalParameters  DVariant=Disabled  IntegratorVariant=Discrete  SatVariant=Disabled  AWVariant=Passthrough  PCopyVariant=Disabled  TRVariant=Disabled  FdbkBlocksVariant=Forward  IdealPFdbkVariant=Disabled  SatFdbkVariant=Disabled  DerivativeFilterVariant=Disabled  NVariant=Disabled  NCopyVariant=Disabled_SignalSpec  FilterICVariant=Disabled  IntegratorICVariant=InternalICs  ExternalResetVariant=Disabled  TRSumVariant=Passthrough  SumFdbkVariant=Disabled  SumVariant=Sum_PI
  Product{,1..4} (5 alike) : Product
  Rf : Constant  Value=0.57
  Sum : Sum  Inputs=|+-
  Sum1 : Sum  Inputs=|+-
  Vd : Outport
  Vq : Outport  Port=2
  wires:
  Idr/1 -> Sum/1
  Idm/1 -> Product/1, Product4/1, Sum/2
  Iqr/1 -> Sum1/1
  Iqm/1 -> Product3/1, Sum1/2
  Sum/1 -> PID Controller/1
  Sum1/1 -> PID Controller1/1
  Gain3/1 -> Vq/1
  Add/1 -> Delay/1
  Vdm/1 -> Add/1
  Product/1 -> Add/3
  Rf/1 -> Gain/1
  Gain/1 -> Product1/2, Product/2
  Lf/1 -> Gain1/1
  PID Controller/1 -> Product1/1
  Product1/1 -> Add/2
  PID Controller1/1 -> Product2/1
  Gain1/1 -> Product4/2, Product3/2, Product2/2
  Gain2/1 -> Vd/1
  Add1/1 -> Delay1/1
  Vqm/1 -> Add1/2
  Product3/1 -> Add1/3, Add/4
  Product2/1 -> Add1/1
  Product4/1 -> Add1/4
  Delay/1 -> Gain2/1
  Delay1/1 -> Gain3/1

== matlab function Modelo_MV_CIGRE_IPSD/DER/Control IBRs/Outer Loop ==
  data: Pr input; Idr output; Qr input; Vd input; Vq input; Ilim input; Iqr output
function [Idr, Iqr] = fcn(Pr,Qr,Vd,Vq,Ilim)

    Id=(Pr*Vd+Qr*Vq)/(Vd^2+Vq^2);
    Iqr=(Pr*Vq-Qr*Vd)/(Vd^2+Vq^2);
    
    if Iqr>Ilim
        Iqr=Ilim*0.95;
    elseif Iqr<-Ilim
        Iqr=-Ilim*0.95;
    end

    Idmax2=Ilim^2-Iqr^2;
    
    if Idmax2<0.01
        Idmax=0;
    else
        Idmax=sqrt(Idmax2);
    end
    
    if and(Id<=Idmax, Id>=-Idmax)
        Idr=Id;
    else 
        Idr=Idmax;
    end
    
    if abs(Idr)<=abs(Idmax)
        Idr=Idr;
    elseif Idr>Idmax
        Idr=Idmax;
    elseif Idr<-Idmax
        Idr=-Idmax;
    end
        
    
    
end

== matlab function Modelo_MV_CIGRE_IPSD/DER/Control IBRs/Ilim ==
  data: Pmax output; v input; Iqmin output; Pr input; Qr input; Ilim input; Pava input
function [Pmax,Iqmin] = fcn(v,Pr,Qr,Ilim,Pava)
    Pmax=Pr;
    
    if v<=0.5
        if abs(Qr)<Ilim*0.9
           Iqmin=Ilim*0.95;
        else
           Iqmin=abs(Qr);
        end
    elseif or(v>0.5,v<=0.85)
            if abs(Qr)<(-18/7*v+153/70)*Ilim
                Iqmin=(-18/7*v+153/70)*Ilim;
            else
                Iqmin=abs(Qr);
            end
    elseif or(v>0.85, v<=0.9)
        if Qr<0
                Iqmin=0;
            else
                Iqmin=Qr;
        end
    else
        Iqmin=abs(Qr);
    end
    
    if v<=0.85
        Idmax=sqrt(abs(Ilim)^2-abs(Iqmin)^2);
    else
        Idmax=1;
    end
   
    if Idmax>Pava
        if Pava>Pr
            Pmax=Pr;
        elseif Idmax>Pr
            Pmax=Pava;
        end
    elseif Pava>Idmax
        if Idmax>Pr
            Pmax=Pr;
        elseif Pava>Pr
            Pmax=Idmax;
        end
    elseif Pr>Pava
        if Pava>Idmax
            Pmax=Idmax;
        elseif Idmax>Pava
            Pmax=Pava;
        end
    end            

end

== matlab function Modelo_MV_CIGRE_IPSD/Bus DER/Gen1 ==
  data: V input; y output; I input; Th_v input; Th_i input; ag output
function [y,ag] = Prot_Gen(V,I,Th_v,Th_i)
    ag=1;
    Vth=0.9;
    Ith=1.1;
    if or(and(I>Ith,V<Vth),V<Vth)
        Th_rf=Th_v-Th_i;
        if or(Th_rf>=90,Th_rf<=-90)
            y=-1; %%Falla atras
        else
            y=1; %%Falla adelante
        end
    else
        Th_r=Th_v-Th_i;
        y=0; %% No falla
    end
end

== matlab function Modelo_MV_CIGRE_IPSD/Bus DER/Carga 1 ==
  data: V input; y output; I input; Th_v input; Th_i input; Th_r input; ag output; I_pf input
function [y,ag] = Prot_Carga(V,I,Th_v,Th_i,Th_r,I_pf)
    ag=3;
    Vth=0.9;
    Ith=1.1;
    if or(and(I>Ith,V<Vth),and(V<Vth,I_pf-I<0))
        Th_rf=Th_v-Th_i;
        if abs(Th_rf-Th_r)<5
            y=0; %%No falla
        else
            if or(Th_rf>=90,Th_rf<=-90)
                y=-1; %%Falla atras
            else
                y=1; %%Falla adelante
            end
        end
    else
        y=0; %% No falla
    end
end

== matlab function Modelo_MV_CIGRE_IPSD/Bus DER/Carga 2 ==
  data: V input; y output; I input; Th_v input; Th_i input; Th_r input; ag output; I_pf input
function [y,ag] = Prot_Carga(V,I,Th_v,Th_i,Th_r,I_pf)
    ag=2;
    Vth=0.9;
    Ith=1.1;
    if or(and(I>Ith,V<Vth),and(V<Vth,I_pf-I<0))
        Th_rf=Th_v-Th_i;
        if abs(Th_rf-Th_r)<5
            y=0; %%No falla
        else
            if or(Th_rf>=90,Th_rf<=-90)
                y=-1; %%Falla atras
            else
                y=1; %%Falla adelante
            end
        end
    else
        y=0; %% No falla
    end
end

== matlab function Modelo_MV_CIGRE_IPSD/Bus DER/MATLAB Function2 ==
  data: V input; Th_r output; I input; Th_v input; Th_i input; Th_r input; I_r input; I_r output
function [Th_r,I_r] = Calc_Ang(V,I,Th_v,Th_i,Th_r,I_r)
    Ith=1.1;
    Vth=0.99;
    if or(and(I<Ith,V>=Vth),V>=Vth)
        Th_r=Th_v-Th_i;
        I_r=I;
    else
        Th_r=Th_r;
        I_r=I_r;
    end
end

== matlab function Modelo_MV_CIGRE_IPSD/Bus DER/Carga 3 ==
  data: V input; y output; I input; Th_v input; Th_i input; Th_r input; ag output; I_pf input
function [y,ag] = Prot_Carga(V,I,Th_v,Th_i,Th_r,I_pf)
    ag=3;
    Vth=0.9;
    Ith=1.1;
    if or(and(I>Ith,V<Vth),V<Vth)
        Th_rf=Th_v-Th_i;
        if abs(Th_rf-Th_r)<1
            y=0; %%No falla
        else
            if or(Th_rf>=90,Th_rf<=-90)
                y=-1; %%Falla atras
            else
                y=1; %%Falla adelante
            end
        end
    else
        y=0; %% No falla
    end
end

== matlab function Modelo_MV_CIGRE_IPSD/Bus DER/MATLAB Function3 ==
  data: V input; Th_r output; I input; Th_v input; Th_i input; Th_r input; I_r input; I_r output
function [Th_r,I_r] = Calc_Ang(V,I,Th_v,Th_i,Th_r,I_r)
    Ith=1.1;
    Vth=0.99;
    if or(and(I<Ith,V>=Vth),V>=Vth)
        Th_r=Th_v-Th_i;
        I_r=I;
    else
        Th_r=Th_r;
        I_r=I_r;
    end
end

== matlab function Modelo_MV_CIGRE_IPSD/Bus PCC/MATLAB Function ==
  data: V input; I_th output; I input; I_th input
function I_th  = I_pickup(V,I,I_th)
% Modificación de la corriente de pickup en función de la corriente de
% carga
    
    Vth=0.9;
    k=1.4;
    if(V>=Vth)
        I_th=1.2*I;
    else
        I_th=I_th;
    end

end

== matlab function Modelo_MV_CIGRE_IPSD/Bus DER/Optim_OP ==
  data: y1 input; y2 input; y3 input; y4 input; tout output; flag input
function tout = optim_operacion(y1,y2,y3,y4,flag)
    CTI=0.1;
    yt=[y1 y2 y3 y4];
    tout=ones(1,length(yt))*10000;
    p=0;
    if flag>0 %%se verifica que se mantengan las condiciones de falla
        top=ones(1,length(yt))*10000;
        A=zeros(length(yt),length(yt));
        C=zeros(length(yt),length(yt));
        for i=1:length(A)
            if yt(i)==1
                p=i;
                C(i,i)=yt(i);
            else
                A(i,i)=yt(i);
                C(i,i)=yt(i);
            end                
        end
        if p~=0
            for i=1:length(A)
                if A(i,i)==-1
                    A(i,p)=1;
                end
            end
        end
        
        j=1;
        B=ones(rank(A),length(yt));
        for i=1:length(A)
            if A(i,i)==-1
                B(j,:)=A(i,:);
                j=j+1;
            end
        end
        if rank(C)==1
            if dot(yt,ones(1,4))==1
                top(1,p)=0.04;
            elseif dot(yt,ones(1,4))==-1
                for i=1:length(yt)
                    if yt(i)==-1
                        top(1,i)=0.1;
                    end
                end
            end
        else
        h=2;
        if p==0
            for i=1:length(yt)
                    if yt(i)==-1
                        top(1,i)=0.1;
                    end
            end
        else
        top(1,p)=0.04;
        while h~=1
            for i=1:length(yt)
                if yt(i)==-1
                    top(1,i)=top(1,p)+0.1;
                end
            end
            Rest=B*top';
            if Rest<=-CTI
                h=1;
            else
                h=2;
            end
        end
        end
        end
    else
        top=ones(1,length(yt))*10000;
    end
    tout=top;
end

== stateflow chart Modelo_MV_CIGRE_IPSD/Bus DER/Chart ==
  state Init
  state No_estable
    out=0
    y=flag
    on after(0.02,sec):
    y1=flag
  state Estable
    out=1
  (default) -> Init
  Init -> No_estable : [even==1]
  No_estable -> Estable : [y1==y && flag~=0]
  data: flag input; out output double; y local double; y1 local double; even input

== matlab function Modelo_MV_CIGRE_IPSD/DER1/Control IBRs/Ilim ==
  data: Pmax output; v input; Iqmin output; Pr input; Qr input; Ilim input; Pava input
function [Pmax,Iqmin] = fcn(v,Pr,Qr,Ilim,Pava)
    Pmax=Pr;
    
    if v<=0.5
        if abs(Qr)<Ilim*0.9
           Iqmin=Ilim*0.95;
        else
           Iqmin=abs(Qr);
        end
    elseif or(v>0.5,v<=0.85)
            if abs(Qr)<(-18/7*v+153/70)*Ilim
                Iqmin=(-18/7*v+153/70)*Ilim;
            else
                Iqmin=abs(Qr);
            end
    elseif or(v>0.85, v<=0.9)
        if Qr<0
                Iqmin=0;
            else
                Iqmin=Qr;
        end
    else
        Iqmin=abs(Qr);
    end
    
    if v<=0.85
        Idmax=sqrt(abs(Ilim)^2-abs(Iqmin)^2);
    else
        Idmax=1;
    end
   
    if Idmax>Pava
        if Pava>Pr
            Pmax=Pr;
        elseif Idmax>Pr
            Pmax=Pava;
        end
    elseif Pava>Idmax
        if Idmax>Pr
            Pmax=Pr;
        elseif Pava>Pr
            Pmax=Idmax;
        end
    elseif Pr>Pava
        if Pava>Idmax
            Pmax=Idmax;
        elseif Idmax>Pava
            Pmax=Pava;
        end
    end            

end

== matlab function Modelo_MV_CIGRE_IPSD/DER1/Control IBRs/Outer Loop ==
  data: Pr input; Idr output; Qr input; Vd input; Vq input; Ilim input; Iqr output
function [Idr, Iqr] = fcn(Pr,Qr,Vd,Vq,Ilim)

    Id=(Pr*Vd+Qr*Vq)/(Vd^2+Vq^2);
    Iqr=(Pr*Vq-Qr*Vd)/(Vd^2+Vq^2);
    
    if Iqr>Ilim
        Iqr=Ilim*0.95;
    elseif Iqr<-Ilim
        Iqr=-Ilim*0.95;
    end

    Idmax2=Ilim^2-Iqr^2;
    
    if Idmax2<0.01
        Idmax=0;
    else
        Idmax=sqrt(Idmax2);
    end
    
    if and(Id<=Idmax, Id>=-Idmax)
        Idr=Id;
    else 
        Idr=Idmax;
    end
    
    if abs(Idr)<=abs(Idmax)
        Idr=Idr;
    elseif Idr>Idmax
        Idr=Idmax;
    elseif Idr<-Idmax
        Idr=-Idmax;
    end
        
    
    
end

== matlab function Modelo_MV_CIGRE_IPSD/Bus PCC/Carga 1 ==
  data: V input; y output; I input; Th_v input; Th_i input; Th_r input; ag output; I_pf input; Ith input
function [y,ag] = Prot_Carga(V,I,Th_v,Th_i,Th_r,I_pf,Ith)
    ag=2;
    Vth=0.9;
    if or(and(I>Ith,V<Vth),and(V<Vth,I_pf-I<0))
        Th_rf=Th_v-Th_i;
        if abs(Th_rf-Th_r)<5
            y=0; %%No falla
        else
            if or(Th_rf>=90,Th_rf<=-90)
                y=-1; %%Falla atras
            else
                y=1; %%Falla adelante
            end
        end
    else
        y=0; %% No falla
    end
end

== stateflow chart Modelo_MV_CIGRE_IPSD/Bus PCC/Chart ==
  state Init
  state No_estable
    out=0
    y=flag
    on after(0.02,sec):
    y1=flag
  state Estable
    out=1
  (default) -> Init
  Init -> No_estable : [even==1]
  No_estable -> Estable : [y1==y && flag~=0]
  data: flag input; out output double; y local double; y1 local double; even input

== matlab function Modelo_MV_CIGRE_IPSD/Bus DER/Optim_OP1 ==
  data: y1 input; y2 input; y3 input; y4 input; y5 input; tout output; flag input; ag_type input; ext input
function tout = optim_operacion(y1,y2,y3,y4,y5,flag, ag_type,ext)
    CTI=0.1;
    yt=[y1 y2 y3 y4 y5];
    tout=ones(1,length(yt))*10000;  
    p=0;
    if flag>0 %%se verifica que se mantengan las condiciones de falla
        top=ones(1,length(yt))*10000;        
        A=zeros(length(yt),length(yt));
        C=zeros(length(yt),length(yt));
        for i=1:length(A) %creación de matrices de coordinación
            if yt(i)==1
                p=i; % se guarda donde se encuentra una falla adelante (solo para eventos unicos)
                C(i,i)=yt(i); 
            else % se crea matriz de coordinación
                A(i,i)=yt(i);
                C(i,i)=yt(i);
            end                
        end
        if p~=0
            for i=1:length(A)
                if A(i,i)==-1
                    A(i,p)=1;
                end
            end
        end
        
        j=1;
        B=ones(rank(A),length(yt));
        for i=1:length(A) %extracción de equipos de respaldo
            if A(i,i)==-1
                B(j,:)=A(i,:);
                j=j+1;
            end
        end
        if rank(C)==1   %verificación de operación individual por equipo
            if dot(yt,ones(1,5))==1
                switch ag_type(p)   %Operación dependiente del tipo de agente
                    case 1
                        top(1,p)=0.04;
                    case 2
                        top(1,p)=0.04;
                    case 3
                        if(yt(p)*ext(p)==1)
                            top(1,p)=0.04;
                        end
                    otherwise
                        top(1,p)=10000;
                end
            elseif dot(yt,ones(1,5))==-1    %Equipos solo en operación de bkup
                for i=1:length(yt)
                        if yt(i)==--1
                            top(1,i)=0.35;
                        end
                end
            end
        else    %Es necesaria la coordinación
        h=2;
        if p==0     % No hay equipo primario al interior del bus
            for i=1:length(yt)
                if yt(i)==-1
                   top(1,i)=0.35;
                end
            end
        else
        switch ag_type(p)
            case 1
               top(1,p)=0.04;
            case 2
                top(1,p)=0.04;
            case 3 
                top(1,p)=0.14;
            otherwise
                top(1,p)=1000;
        end
        
        while h~=1
            for i=1:length(yt)
                if yt(i)==-1
                    top(1,i)=top(1,p)+0.1;
                end
            end
            Rest=B*top';
            if Rest<=-CTI
                h=1;
            else
                h=2;
            end
        end
        end
        end
    else
        top=ones(1,length(yt))*10000;
    end
    tout=top;
end

== matlab function Modelo_MV_CIGRE_IPSD/Bus PCC/Carga 2 ==
  data: V input; y output; I input; Th_v input; Th_i input; Th_r input; ag output; I_pf input
function [y,ag] = Prot_Carga(V,I,Th_v,Th_i,Th_r,I_pf)
    ag=3;
    Vth=0.9;
    Ith=1.1;
    if or(and(I>Ith,V<Vth),and(V<Vth,I_pf-I<0))
        Th_rf=Th_v-Th_i;
        if abs(Th_rf-Th_r)<5
            y=0; %%No falla
        else
            if or(Th_rf>=90,Th_rf<=-90)
                y=-1; %%Falla atras
            else
                y=1; %%Falla adelante
            end
        end
    else
        y=0; %% No falla
    end
end

== matlab function Modelo_MV_CIGRE_IPSD/Bus PCC/Carga 3 ==
  data: V input; y output; I input; Th_v input; Th_i input; Th_r input; ag output; I_pf input
function [y,ag] = Prot_Carga(V,I,Th_v,Th_i,Th_r,I_pf)
    ag=3;
    Vth=0.9;
    Ith=1.1;
    if or(and(I>Ith,V<Vth),and(V<Vth,I_pf-I<0))
        Th_rf=Th_v-Th_i;
        if abs(Th_rf-Th_r)<5
            y=0; %%No falla
        else
            if or(Th_rf>=90,Th_rf<=-90)
                y=-1; %%Falla atras
            else
                y=1; %%Falla adelante
            end
        end
    else
        y=0; %% No falla
    end
end

== matlab function Modelo_MV_CIGRE_IPSD/Bus PCC/MATLAB Function2 ==
  data: V input; Th_r output; I input; Th_v input; Th_i input; Th_r input; I_r input; I_r output; Ith input
function [Th_r,I_r] = Calc_Ang(V,I,Th_v,Th_i,Th_r,I_r, Ith)
    Vth=0.99;
    if or(and(I<Ith,V>=Vth),V>=Vth)
        Th_r=Th_v-Th_i;
        I_r=I;
    else
        Th_r=Th_r;
        I_r=I_r;
    end
end

== matlab function Modelo_MV_CIGRE_IPSD/Bus DER/MATLAB Function1 ==
  data: V input; Th_r output; I input; Th_v input; Th_i input; Th_r input; I_r input; I_r output
function [Th_r,I_r] = Calc_Ang(V,I,Th_v,Th_i,Th_r,I_r)
    Ith=1.1;
    Vth=0.99;
    if or(and(I<Ith,V>=Vth),V>=Vth)
        Th_r=Th_v-Th_i;
        I_r=I;
    else
        Th_r=Th_r;
        I_r=I_r;
    end
end

== matlab function Modelo_MV_CIGRE_IPSD/Bus PCC/MATLAB Function6 ==
  data: V input; Th_r output; I input; Th_v input; Th_i input; Th_r input; I_r input; I_r output
function [Th_r,I_r] = Calc_Ang(V,I,Th_v,Th_i,Th_r,I_r)
    Ith=1.1;
    Vth=0.99;
    if or(and(I<Ith,V>=Vth),V>=Vth)
        Th_r=Th_v-Th_i;
        I_r=I;
    else
        Th_r=Th_r;
        I_r=I_r;
    end
end

== matlab function Modelo_MV_CIGRE_IPSD/Bus9_UA/Carga 2 ==
  data: V input; y output; I input; Th_v input; Th_i input; Th_r input; I_pf input
function y = Prot_Carga(V,I,Th_v,Th_i,Th_r,I_pf)
    ag=2;
    Vth=0.9;
    Ith=1.1;
    if or(V<Vth)
        Th_rf=Th_v-Th_i;
        if abs(Th_rf-Th_r)<2
            y=0; %%No falla
        else
            if or(Th_rf>=90,Th_rf<=-90)
                y=-1; %%Falla atras
            else
                y=1; %%Falla adelante
            end
        end
    else
        y=0; %% No falla
    end
end
